simulink model "F550_waypoint"  (R2024a)
settings: Solver=ode4  StartTime=0.0  StopTime=50  FixedStep=Ts  RelTol=1e-3
values from neighbouring files (symbols this model uses):
  armLength = 0.275    [F550_data.m]
  Cd = 0.055    [F550_data.m]
  Cmd = [0.0035 0.0039 0.0034]    [F550_data.m]
  dzcg = 0.12    [F550_data.m]
  g = 9.81    [F550_data.m]
  Inertia = [Jxx, 0, 0;     0, Jyy, 0;     0, 0, Jzz]    [F550_data.m]
  Inertia_inv = inv(Inertia)    [F550_data.m]
  Kd_theta = 1    [sim_F550_waypoint.m]
  Ki_h = 0    [sim_F550_waypoint.m]
  Ki_psi = 0    [sim_F550_waypoint.m]
  Ki_u = 0.02    [sim_F550_waypoint.m]
  Ki_vs = 0.01    [sim_F550_waypoint.m]
  Kp_h = 0.1    [sim_F550_waypoint.m]
  Kp_psi = 1.6    [sim_F550_waypoint.m]
  Kp_r = 0.15    [sim_F550_waypoint.m]
  Kp_theta = 5    [sim_F550_waypoint.m]
  Kp_u = 0.2    [sim_F550_waypoint.m]
  Kp_vs = 0.1    [sim_F550_waypoint.m]
  Mass = 2.06    [F550_data.m]
  motorCr = 1148    [F550_data.m]
  motorJm = 0.0001287    [F550_data.m]
  motorRpm0 = [4000 4000 4000 4000 4000 4000]    [F550_data.m]
  motorTm = 0.02    [F550_data.m]
  motorWb = -141.4    [F550_data.m]
  rotorCm = 1.779e-07    [F550_data.m]
  rotorCt = 1.105e-05    [F550_data.m]
  u0 = opreport.inputs.u    [trim_F550_model.m]
  wp_alt = [100 120 150  80  80]    [sim_F550_waypoint.m]
  wp_east = [0   400 500 500   0]    [sim_F550_waypoint.m]
  wp_north = [100 100 300 500 300]    [sim_F550_waypoint.m]
  wp_u = [  3   5   5   4   3]    [sim_F550_waypoint.m]
  x0 = [0 0 0 0 0 0 0 0 0 0 0 -500]    [F550_data.m]    (also in trim_F550_model.m = opreport.states(7).x)
libraries: matrix_library x2
settings Model: Creator=ADMIN  LastModifiedBy=CNU_UASG
settings DataIOCC: ReturnWorkspaceOutputs=off
settings DebuggingCC: UnconnectedInputMsg=warning  UnconnectedOutputMsg=warning  UnconnectedLineMsg=warning
settings ModelReferenceCC: EnableRefExpFcnMdlSchedulingChecks=on
settings RTWCC: GPUComputeCapability=3.5  DLArmComputeVersion=19.05

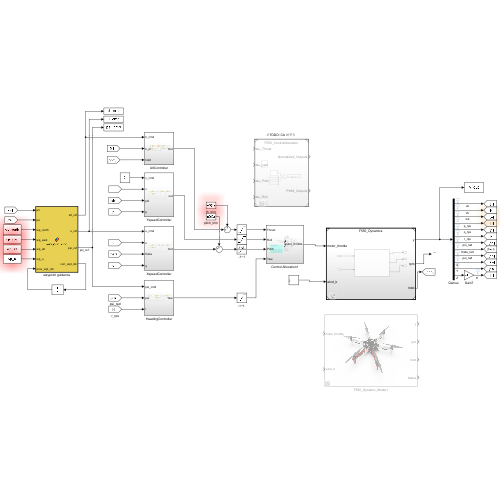
[thumbnail: Simulink's stored preview of the top-level diagram]
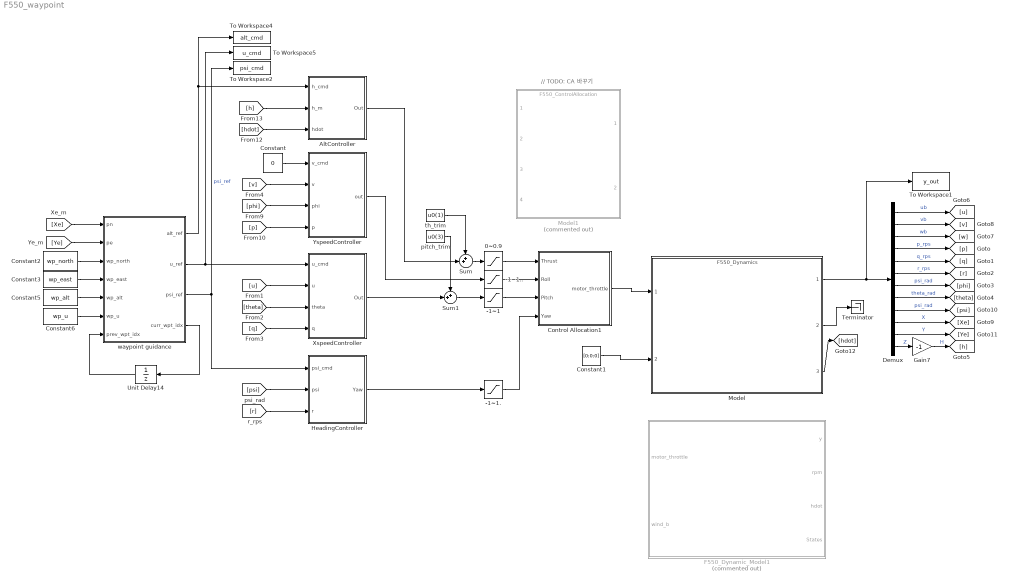
== system F550_waypoint ==
  note: // TODO: CA 바꾸기
  -1~1 : Saturate  UpperLimit=1  LowerLimit=-1
  -1~1. : Saturate  UpperLimit=1  LowerLimit=-1
  -1~1.. : Saturate  UpperLimit=1  LowerLimit=-1
  0~0.9 : Saturate  UpperLimit=0.9  LowerLimit=0
  AltController : Subsystem
  Constant : Constant  Value=0
  Constant1 : Constant  Value=[0;0;0]
  Constant2 : Constant  Value=wp_north  OutDataTypeStr=double
  Constant3 : Constant  Value=wp_east  OutDataTypeStr=double
  Constant5 : Constant  Value=wp_alt  OutDataTypeStr=double
  Constant6 : Constant  Value=wp_u  OutDataTypeStr=double
  Control Allocation1 : Subsystem
  Demux : Demux  Outputs=12
  F550_Dynamic_Model1 : Subsystem  Commented=on
      mask Display: image('F550.jpg');
  Gain7 : Gain  Gain=-1
  HeadingController : Subsystem
  Model : ModelReference  ModelNameDialog=F550_Dynamics.slx  SimulationMode=Normal  ModelReferenceVersion=1.4
  Model1 : ModelReference  Commented=on  ModelNameDialog=F550_ControlAllocation.slx  SimulationMode=Normal  ModelReferenceVersion=1.2
  Sum : Sum  Inputs=++|
  Sum1 : Sum  Inputs=++|
  Terminator : Terminator
  To Workspace1 : ToWorkspace  VariableName=y_out  SampleTime=-1
  To Workspace2 : ToWorkspace  VariableName=psi_cmd  SampleTime=-1
  To Workspace4 : ToWorkspace  VariableName=alt_cmd  SampleTime=-1
  To Workspace5 : ToWorkspace  VariableName=u_cmd  SampleTime=-1
  Unit Delay14 : UnitDelay  InitialCondition=1  SampleTime=-1  HasFrameUpgradeWarning=on
  XspeedController : Subsystem
  YspeedController : Subsystem
  pitch_trim : Constant  Value=u0(3)  OutDataTypeStr=double
  th_trim : Constant  Value=u0(1)  OutDataTypeStr=double
  waypoint guidance : MATLAB Function  TreatAsAtomicUnit=on
  wires:
  th_trim/1 -> Sum/1
  AltController/1(Out) -> Sum/2
  Sum/1 -> 0~0.9/1
  YspeedController/1(out) -> -1~1../1
  Demux/2 -> [v]  "vb"
  Demux/6 -> [r]  "r_rps"
  Demux/8 -> [theta]  "theta_rad"
  Gain7/1 -> [h]  "H"
  Demux/12 -> Gain7/1  "Z"
  Demux/5 -> [q]  "q_rps"
  Demux/3 -> [w]  "wb"
  Demux/4 -> [p]  "p_rps"
  Demux/7 -> [phi]  "psi_rad"
  Demux/1 -> [u]  "ub"
  Model/1 -> To Workspace1/1, Demux/1
  Demux/10 -> [Xe]  "X"
  Demux/11 -> [Ye]  "Y"
  0~0.9/1 -> Control Allocation1/1(Thrust)
  Demux/9 -> [psi]  "psi_rad"
  Constant3/1 -> waypoint guidance/4(wp_east)
  Constant2/1 -> waypoint guidance/3(wp_north)
  waypoint guidance/4(curr_wpt_idx) -> Unit Delay14/1
  Unit Delay14/1 -> waypoint guidance/7(prev_wpt_idx)
  [q] -> XspeedController/4(q)
  [theta] -> XspeedController/3(theta)
  [u] -> XspeedController/2(u)
  waypoint guidance/1(alt_ref) -> AltController/1(h_cmd), To Workspace4/1
  [h] -> AltController/2(h_m)
  [hdot] -> AltController/3(hdot)
  waypoint guidance/3(psi_ref) -> HeadingController/1(psi_cmd), To Workspace2/1  "psi_ref"
  [psi] -> HeadingController/2(psi)
  [r] -> HeadingController/3(r)
  [Ye] -> waypoint guidance/2(pe)
  [Xe] -> waypoint guidance/1(pn)
  Control Allocation1/1(motor_throttle) -> Model/1
  Constant1/1 -> Model/2
  Model/2 -> Terminator/1
  Model/3 -> [hdot]
  Sum1/1 -> -1~1/1
  pitch_trim/1 -> Sum1/1
  XspeedController/1(Out) -> Sum1/2
  -1~1/1 -> Control Allocation1/3(Pitch)
  -1~1./1 -> Control Allocation1/4(Yaw)
  HeadingController/1(Yaw) -> -1~1./1
  Constant/1 -> YspeedController/1(v_cmd)
  [v] -> YspeedController/2(v)
  [phi] -> YspeedController/3(phi)
  [p] -> YspeedController/4(p)
  -1~1../1 -> Control Allocation1/2(Roll)
  Constant5/1 -> waypoint guidance/5(wp_alt)
  Constant6/1 -> waypoint guidance/6(wp_u)
  waypoint guidance/2(u_ref) -> XspeedController/1(u_cmd), To Workspace5/1

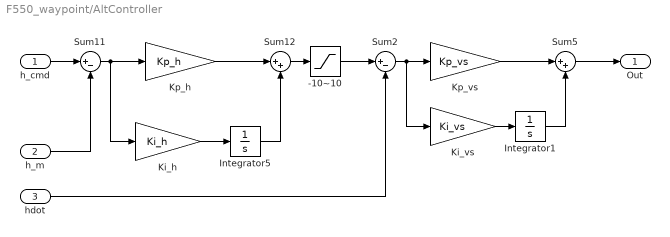
== system F550_waypoint/AltController ==
  h_cmd : Inport
  h_m : Inport  Port=2
  hdot : Inport  Port=3
  -10~10 : Saturate  UpperLimit=10  LowerLimit=-10
  Integrator1 : Integrator
  Integrator5 : Integrator
  Ki_h : Gain  Gain=Ki_h  SaturateOnIntegerOverflow=on  OutDataTypeStr=Inherit: Same as input  ParamDataTypeStr=Inherit: Same as input
  Ki_vs : Gain  Gain=Ki_vs  SaturateOnIntegerOverflow=on  OutDataTypeStr=Inherit: Same as input  ParamDataTypeStr=Inherit: Same as input
  Kp_h : Gain  Gain=Kp_h  SaturateOnIntegerOverflow=on  OutDataTypeStr=Inherit: Same as input  ParamDataTypeStr=Inherit: Same as input
  Kp_vs : Gain  Gain=Kp_vs  SaturateOnIntegerOverflow=on  OutDataTypeStr=Inherit: Same as input  ParamDataTypeStr=Inherit: Same as input
  Sum11 : Sum  Inputs=|+-  InputSameDT=on  SaturateOnIntegerOverflow=on  OutDataTypeStr=Inherit: Same as first input
  Sum12 : Sum  Inputs=|++  InputSameDT=on  SaturateOnIntegerOverflow=on  OutDataTypeStr=Inherit: Same as first input
  Sum2 : Sum  Inputs=|+-  InputSameDT=on  SaturateOnIntegerOverflow=on  OutDataTypeStr=Inherit: Same as first input
  Sum5 : Sum  Inputs=|++  InputSameDT=on  SaturateOnIntegerOverflow=on  OutDataTypeStr=Inherit: Same as first input
  Out : Outport
  wires:
  -10~10/1 -> Sum2/1
  Sum11/1 -> Kp_h/1, Ki_h/1
  Kp_vs/1 -> Sum5/1
  Sum12/1 -> -10~10/1
  Integrator1/1 -> Sum5/2
  Sum2/1 -> Kp_vs/1, Ki_vs/1
  Integrator5/1 -> Sum12/2
  Ki_h/1 -> Integrator5/1
  Kp_h/1 -> Sum12/1
  Ki_vs/1 -> Integrator1/1
  Sum5/1 -> Out/1
  h_m/1 -> Sum11/2
  h_cmd/1 -> Sum11/1
  hdot/1 -> Sum2/2

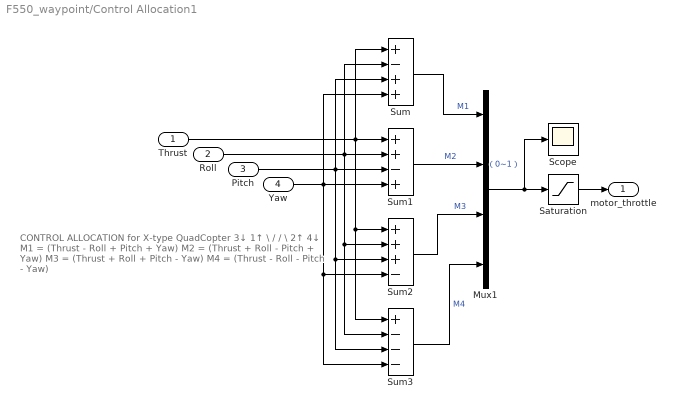
== system F550_waypoint/Control Allocation1 ==
  note: CONTROL ALLOCATION
      | for X-type QuadCopter
      | 3↓ 1↑
      | \ /
      | / \
      | 2↑ 4↓
      | M1 = (Thrust - Roll + Pitch + Yaw)
      | M2 = (Thrust + Roll - Pitch + Yaw)
      | M3 = (Thrust + Roll + Pitch - Yaw)
      | M4 = (Thrust - Roll - Pitch - Yaw)
  Thrust : Inport
  Roll : Inport  Port=2
  Pitch : Inport  Port=3
  Yaw : Inport  Port=4
  Mux1 : Mux
  Saturation : Saturate  UpperLimit=1  LowerLimit=0
  Scope : Scope
  Sum : Sum  Inputs=+-++
  Sum1 : Sum  Inputs=++-+
  Sum2 : Sum  Inputs=+++-
  Sum3 : Sum  Inputs=+---
  motor_throttle : Outport
  wires:
  Thrust/1 -> Sum3/1, Sum2/1, Sum/1, Sum1/1
  Sum3/1 -> Mux1/4  "M4"
  Sum1/1 -> Mux1/2  "M2"
  Yaw/1 -> Sum3/4, Sum2/4, Sum/4, Sum1/4
  Sum/1 -> Mux1/1  "M1"
  Roll/1 -> Sum3/2, Sum2/2, Sum/2, Sum1/2
  Sum2/1 -> Mux1/3  "M3"
  Mux1/1 -> Scope/1, Saturation/1  "（0~1）"
  Pitch/1 -> Sum3/3, Sum2/3, Sum/3, Sum1/3
  Saturation/1 -> motor_throttle/1

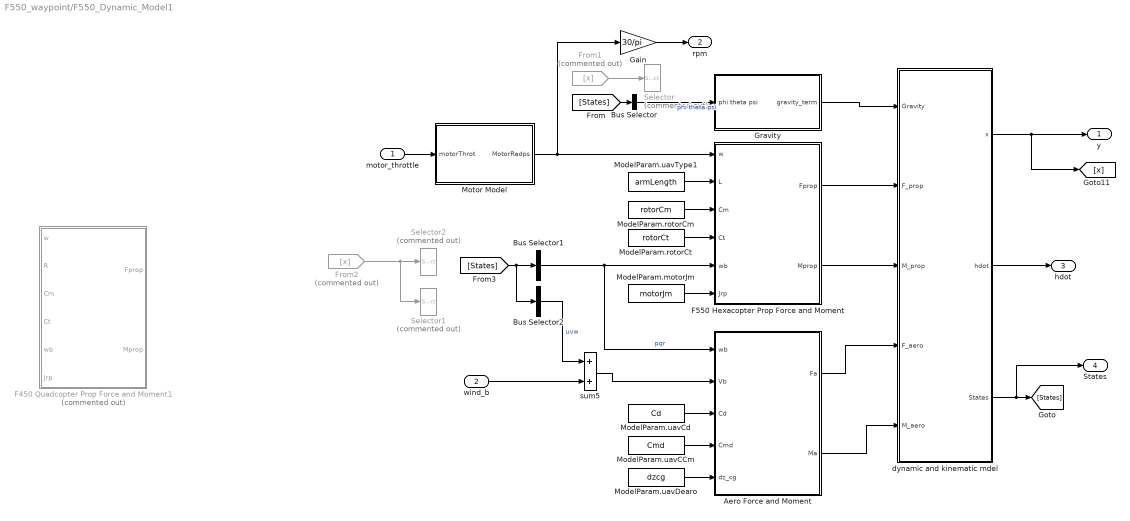
== system F550_waypoint/F550_Dynamic_Model1 ==
  motor_throttle : Inport
  wind_b : Inport  Port=2
  Aero Force and Moment : MATLAB Function  TreatAsAtomicUnit=on
  Bus Selector : BusSelector  OutputSignals=Phi,Theta,Psi  OutputAsBus=on
  Bus Selector1 : BusSelector  OutputSignals=P,Q,R  OutputAsBus=on
  Bus Selector2 : BusSelector  OutputSignals=U,V,W  OutputAsBus=on
  F450 Quadcopter Prop Force and Moment1 : MATLAB Function  Commented=on  TreatAsAtomicUnit=on
  F550 Hexacopter Prop Force and Moment : MATLAB Function  TreatAsAtomicUnit=on
  From1 : From  Commented=on  GotoTag=x
  From2 : From  Commented=on  GotoTag=x
  Gain : Gain  Gain=30/pi
  Gravity : Subsystem
  ModelParam.motorJm : Constant  Value=motorJm
  ModelParam.rotorCm : Constant  Value=rotorCm
  ModelParam.rotorCt : Constant  Value=rotorCt
  ModelParam.uavCCm : Constant  Value=Cmd
  ModelParam.uavCd : Constant  Value=Cd
  ModelParam.uavDearo : Constant  Value=dzcg
  ModelParam.uavType1 : Constant  Value=armLength
  Motor Model : Subsystem
  Selector : Selector  Commented=on  InputPortWidth=12  IndexOptions=Index vector (dialog)  Indices=[7 8 9]  OutputSizes=1
  Selector1 : Selector  Commented=on  InputPortWidth=12  IndexOptions=Index vector (dialog)  Indices=[1 2 3]  OutputSizes=1
  Selector2 : Selector  Commented=on  InputPortWidth=12  IndexOptions=Index vector (dialog)  Indices=[4 5 6]  OutputSizes=1
  dynamic and kinematic mdel : Subsystem
  sum5 : Sum  InputSameDT=on  SaturateOnIntegerOverflow=on  OutDataTypeStr=Inherit: Same as first input
  y : Outport
  rpm : Outport  Port=2
  hdot : Outport  Port=3
  States : Outport  Port=4
  wires:
  ModelParam.uavDearo/1 -> Aero Force and Moment/5(dz_cg)
  ModelParam.uavCCm/1 -> Aero Force and Moment/4(Cmd)
  ModelParam.uavCd/1 -> Aero Force and Moment/3(Cd)
  Aero Force and Moment/2(Ma) -> dynamic and kinematic mdel/5(M_aero)
  Aero Force and Moment/1(Fa) -> dynamic and kinematic mdel/4(F_aero)
  F550 Hexacopter Prop Force and Moment/2(Mprop) -> dynamic and kinematic mdel/3(M_prop)
  F550 Hexacopter Prop Force and Moment/1(Fprop) -> dynamic and kinematic mdel/2(F_prop)
  ModelParam.motorJm/1 -> F550 Hexacopter Prop Force and Moment/6(Jrp)
  ModelParam.uavType1/1 -> F550 Hexacopter Prop Force and Moment/2(L)
  ModelParam.rotorCt/1 -> F550 Hexacopter Prop Force and Moment/4(Ct)
  ModelParam.rotorCm/1 -> F550 Hexacopter Prop Force and Moment/3(Cm)
  Gravity/1(gravity_term) -> dynamic and kinematic mdel/1(Gravity)
  motor_throttle/1 -> Motor Model/1(motorThrot)
  Gain/1 -> rpm/1
  From1/1 -> Selector/1
  From2/1 -> Selector2/1, Selector1/1
  Motor Model/1(MotorRadps) -> F550 Hexacopter Prop Force and Moment/1(w), Gain/1
  wind_b/1 -> sum5/2
  sum5/1 -> Aero Force and Moment/2(Vb)
  dynamic and kinematic mdel/1(x) -> y/1, [x]
  dynamic and kinematic mdel/2(hdot) -> hdot/1
  dynamic and kinematic mdel/3(States) -> States/1, [States]
  [States] -> Bus Selector/1
  Bus Selector/1 -> Gravity/1(phi theta psi)  "phi theta psi"
  [States] -> Bus Selector2/1, Bus Selector1/1
  Bus Selector1/1 -> Aero Force and Moment/1(wb), F550 Hexacopter Prop Force and Moment/5(wb)  "pqr"
  Bus Selector2/1 -> sum5/1  "uvw"

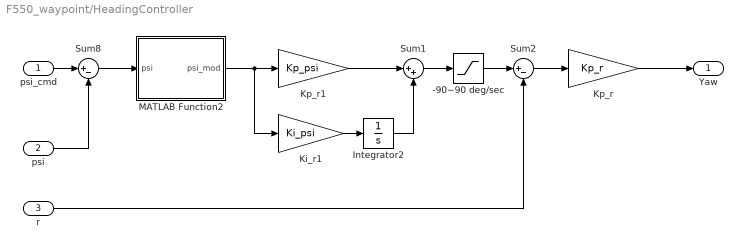
== system F550_waypoint/HeadingController ==
  psi_cmd : Inport
  psi : Inport  Port=2
  r : Inport  Port=3
  -90~90 deg/sec : Saturate  UpperLimit=90/57.3  LowerLimit=-90/57.3
  Integrator2 : Integrator
  Ki_r1 : Gain  Gain=Ki_psi  SaturateOnIntegerOverflow=on  OutDataTypeStr=Inherit: Same as input  ParamDataTypeStr=Inherit: Same as input
  Kp_r : Gain  Gain=Kp_r  SaturateOnIntegerOverflow=on  OutDataTypeStr=Inherit: Same as input  ParamDataTypeStr=Inherit: Same as input
  Kp_r1 : Gain  Gain=Kp_psi  SaturateOnIntegerOverflow=on  OutDataTypeStr=Inherit: Same as input  ParamDataTypeStr=Inherit: Same as input
  MATLAB Function2 : MATLAB Function  TreatAsAtomicUnit=on
  Sum1 : Sum  Inputs=|++  InputSameDT=on  SaturateOnIntegerOverflow=on  OutDataTypeStr=Inherit: Same as first input
  Sum2 : Sum  Inputs=|+-  InputSameDT=on  SaturateOnIntegerOverflow=on  OutDataTypeStr=Inherit: Same as first input
  Sum8 : Sum  Inputs=|+-  InputSameDT=on  SaturateOnIntegerOverflow=on  OutDataTypeStr=Inherit: Same as first input
  Yaw : Outport
  wires:
  Sum2/1 -> Kp_r/1
  Sum1/1 -> -90~90 deg/sec/1
  Kp_r1/1 -> Sum1/1
  Kp_r/1 -> Yaw/1
  Ki_r1/1 -> Integrator2/1
  Integrator2/1 -> Sum1/2
  -90~90 deg/sec/1 -> Sum2/1
  r/1 -> Sum2/2
  psi/1 -> Sum8/2
  psi_cmd/1 -> Sum8/1
  Sum8/1 -> MATLAB Function2/1(psi)
  MATLAB Function2/1(psi_mod) -> Kp_r1/1, Ki_r1/1

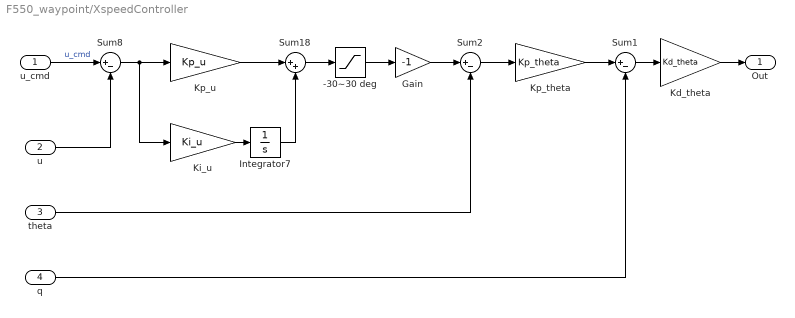
== system F550_waypoint/XspeedController ==
  u_cmd : Inport
  u : Inport  Port=2
  theta : Inport  Port=3
  q : Inport  Port=4
  -30~30 deg : Saturate  UpperLimit=30/57.3  LowerLimit=-30/57.3
  Gain : Gain  Gain=-1
  Integrator7 : Integrator
  Kd_theta : Gain  Gain=Kd_theta  SaturateOnIntegerOverflow=on  OutDataTypeStr=Inherit: Same as input  ParamDataTypeStr=Inherit: Same as input
  Ki_u : Gain  Gain=Ki_u  SaturateOnIntegerOverflow=on  OutDataTypeStr=Inherit: Same as input  ParamDataTypeStr=Inherit: Same as input
  Kp_theta : Gain  Gain=Kp_theta  SaturateOnIntegerOverflow=on  OutDataTypeStr=Inherit: Same as input  ParamDataTypeStr=Inherit: Same as input
  Kp_u : Gain  Gain=Kp_u  SaturateOnIntegerOverflow=on  OutDataTypeStr=Inherit: Same as input  ParamDataTypeStr=Inherit: Same as input
  Sum1 : Sum  Inputs=|+-  InputSameDT=on  SaturateOnIntegerOverflow=on  OutDataTypeStr=Inherit: Same as first input
  Sum18 : Sum  Inputs=|++  InputSameDT=on  SaturateOnIntegerOverflow=on  OutDataTypeStr=Inherit: Same as first input
  Sum2 : Sum  Inputs=|+-  InputSameDT=on  SaturateOnIntegerOverflow=on  OutDataTypeStr=Inherit: Same as first input
  Sum8 : Sum  Inputs=|+-  InputSameDT=on  SaturateOnIntegerOverflow=on  OutDataTypeStr=Inherit: Same as first input
  Out : Outport
  wires:
  -30~30 deg/1 -> Gain/1
  Kp_u/1 -> Sum18/1
  Sum2/1 -> Kp_theta/1
  Ki_u/1 -> Integrator7/1
  Sum18/1 -> -30~30 deg/1
  theta/1 -> Sum2/2
  Sum8/1 -> Ki_u/1, Kp_u/1
  Gain/1 -> Sum2/1
  q/1 -> Sum1/2
  Integrator7/1 -> Sum18/2
  Kp_theta/1 -> Sum1/1
  u_cmd/1 -> Sum8/1  "u_cmd"
  Sum1/1 -> Kd_theta/1
  u/1 -> Sum8/2
  Kd_theta/1 -> Out/1

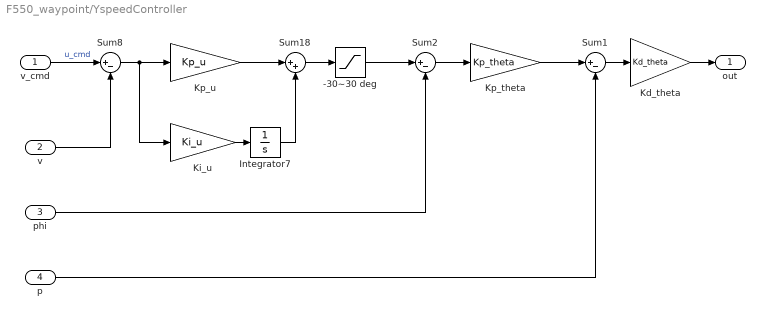
== system F550_waypoint/YspeedController ==
  v_cmd : Inport
  v : Inport  Port=2
  phi : Inport  Port=3
  p : Inport  Port=4
  -30~30 deg : Saturate  UpperLimit=30/57.3  LowerLimit=-30/57.3
  Integrator7 : Integrator
  Kd_theta : Gain  Gain=Kd_theta  SaturateOnIntegerOverflow=on  OutDataTypeStr=Inherit: Same as input  ParamDataTypeStr=Inherit: Same as input
  Ki_u : Gain  Gain=Ki_u  SaturateOnIntegerOverflow=on  OutDataTypeStr=Inherit: Same as input  ParamDataTypeStr=Inherit: Same as input
  Kp_theta : Gain  Gain=Kp_theta  SaturateOnIntegerOverflow=on  OutDataTypeStr=Inherit: Same as input  ParamDataTypeStr=Inherit: Same as input
  Kp_u : Gain  Gain=Kp_u  SaturateOnIntegerOverflow=on  OutDataTypeStr=Inherit: Same as input  ParamDataTypeStr=Inherit: Same as input
  Sum1 : Sum  Inputs=|+-  InputSameDT=on  SaturateOnIntegerOverflow=on  OutDataTypeStr=Inherit: Same as first input
  Sum18 : Sum  Inputs=|++  InputSameDT=on  SaturateOnIntegerOverflow=on  OutDataTypeStr=Inherit: Same as first input
  Sum2 : Sum  Inputs=|+-  InputSameDT=on  SaturateOnIntegerOverflow=on  OutDataTypeStr=Inherit: Same as first input
  Sum8 : Sum  Inputs=|+-  InputSameDT=on  SaturateOnIntegerOverflow=on  OutDataTypeStr=Inherit: Same as first input
  out : Outport
  wires:
  Kd_theta/1 -> out/1
  v/1 -> Sum8/2
  Sum1/1 -> Kd_theta/1
  v_cmd/1 -> Sum8/1  "u_cmd"
  Kp_theta/1 -> Sum1/1
  Integrator7/1 -> Sum18/2
  p/1 -> Sum1/2
  Sum8/1 -> Kp_u/1, Ki_u/1
  phi/1 -> Sum2/2
  Sum18/1 -> -30~30 deg/1
  Ki_u/1 -> Integrator7/1
  Sum2/1 -> Kp_theta/1
  Kp_u/1 -> Sum18/1
  -30~30 deg/1 -> Sum2/1

== system F550_waypoint/F550_Dynamic_Model1/Gravity ==
  note: Gravaity
  phi theta psi : Inport
  . : Gain  Gain=g*Mass  SaturateOnIntegerOverflow=on  OutDataTypeStr=Inherit: Same as input  ParamDataTypeStr=Inherit: Same as input
  Mux : Mux  Inputs=3
  psidot2 : Fcn  Expr=cos(u[2])*cos(u[1])
  t : Fcn  Expr=-sin(u[2])
  tetadot : Fcn  Expr=cos(u[2])*sin(u[1])
  gravity_term : Outport  InitialOutput=0  VectorParamsAs1DForOutWhenUnconnected=off
  wires:
  t/1 -> Mux/1
  psidot2/1 -> Mux/3
  tetadot/1 -> Mux/2
  Mux/1 -> ./1
  phi theta psi/1 -> tetadot/1, t/1, psidot2/1
  ./1 -> gravity_term/1

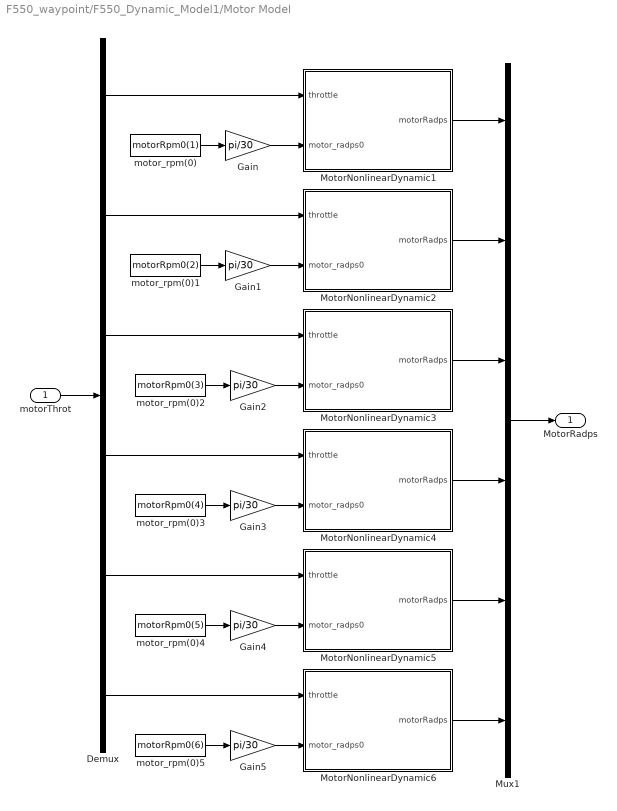
== system F550_waypoint/F550_Dynamic_Model1/Motor Model ==
  motorThrot : Inport
  Demux : Demux  Outputs=6
  Gain{,1..5} (6 alike) : Gain  Gain=pi/30
  MotorNonlinearDynamic1 : Subsystem  TreatAsAtomicUnit=on
  MotorNonlinearDynamic2 : Subsystem  TreatAsAtomicUnit=on
  MotorNonlinearDynamic3 : Subsystem  TreatAsAtomicUnit=on
  MotorNonlinearDynamic4 : Subsystem  TreatAsAtomicUnit=on
  MotorNonlinearDynamic5 : Subsystem  TreatAsAtomicUnit=on
  MotorNonlinearDynamic6 : Subsystem  TreatAsAtomicUnit=on
  Mux1 : Mux  Inputs=6
  motor_rpm(0) : Constant  Value=motorRpm0(1)
  motor_rpm(0)1 : Constant  Value=motorRpm0(2)
  motor_rpm(0)2 : Constant  Value=motorRpm0(3)
  motor_rpm(0)3 : Constant  Value=motorRpm0(4)
  motor_rpm(0)4 : Constant  Value=motorRpm0(5)
  motor_rpm(0)5 : Constant  Value=motorRpm0(6)
  MotorRadps : Outport  VectorParamsAs1DForOutWhenUnconnected=off
  wires:
  motorThrot/1 -> Demux/1
  Demux/4 -> MotorNonlinearDynamic4/1(throttle)
  motor_rpm(0)/1 -> Gain/1
  MotorNonlinearDynamic3/1(motorRadps) -> Mux1/3
  MotorNonlinearDynamic2/1(motorRadps) -> Mux1/2
  Mux1/1 -> MotorRadps/1
  Demux/2 -> MotorNonlinearDynamic2/1(throttle)
  Demux/3 -> MotorNonlinearDynamic3/1(throttle)
  Demux/1 -> MotorNonlinearDynamic1/1(throttle)
  MotorNonlinearDynamic4/1(motorRadps) -> Mux1/4
  MotorNonlinearDynamic1/1(motorRadps) -> Mux1/1
  Gain/1 -> MotorNonlinearDynamic1/2(motor_radps0)
  motor_rpm(0)1/1 -> Gain1/1
  Gain1/1 -> MotorNonlinearDynamic2/2(motor_radps0)
  motor_rpm(0)2/1 -> Gain2/1
  Gain2/1 -> MotorNonlinearDynamic3/2(motor_radps0)
  motor_rpm(0)3/1 -> Gain3/1
  Gain3/1 -> MotorNonlinearDynamic4/2(motor_radps0)
  Gain4/1 -> MotorNonlinearDynamic5/2(motor_radps0)
  motor_rpm(0)4/1 -> Gain4/1
  Demux/5 -> MotorNonlinearDynamic5/1(throttle)
  Gain5/1 -> MotorNonlinearDynamic6/2(motor_radps0)
  motor_rpm(0)5/1 -> Gain5/1
  Demux/6 -> MotorNonlinearDynamic6/1(throttle)
  MotorNonlinearDynamic5/1(motorRadps) -> Mux1/5
  MotorNonlinearDynamic6/1(motorRadps) -> Mux1/6

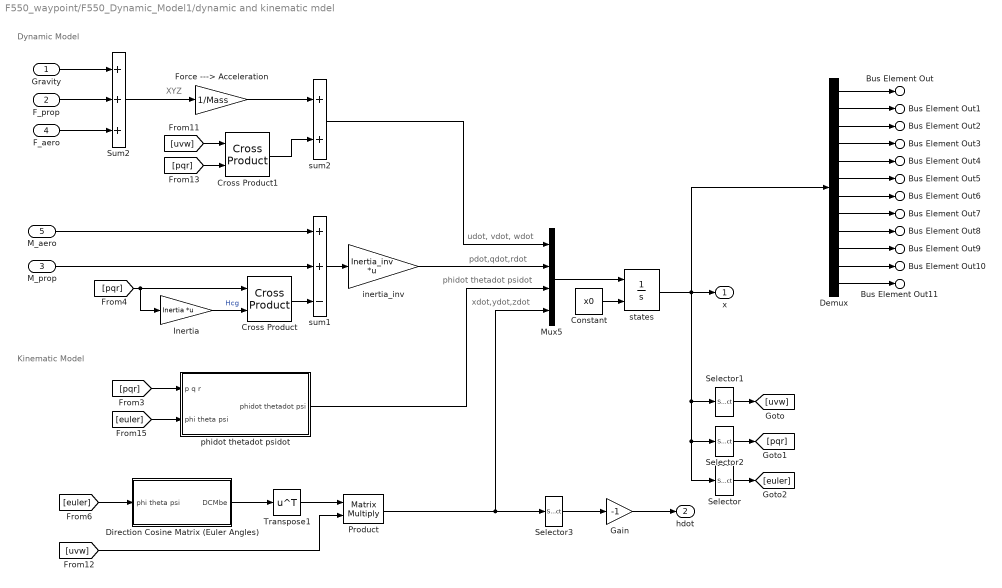
== system F550_waypoint/F550_Dynamic_Model1/dynamic and kinematic mdel ==
  note: Kinematic Model
  note: udot, vdot, wdot
  note: pdot,qdot,rdot
  note: phidot thetadot psidot
  note: xdot,ydot,zdot
  note: XYZ
  note: Dynamic Model
  Gravity : Inport
  F_prop : Inport  Port=2
  M_prop : Inport  Port=3
  F_aero : Inport  Port=4
  M_aero : Inport  Port=5
  Constant : Constant  Value=x0
  Cross Product : matrix_library/Cross Product
  Cross Product1 : matrix_library/Cross Product
  Demux : Demux  Outputs=12
  Direction Cosine Matrix (Euler Angles) : Subsystem
  Force ---> Acceleration : Gain  Gain=1/Mass  SaturateOnIntegerOverflow=on  OutDataTypeStr=Inherit: Same as input  ParamDataTypeStr=Inherit: Same as input
  Gain : Gain  Gain=-1
  Inertia : Gain  Gain=Inertia  Multiplication=Matrix(K*u)
  Mux5 : Mux
  Product : Product  Multiplication=Matrix(*)  InputSameDT=on  RndMeth=Zero  SaturateOnIntegerOverflow=on  OutDataTypeStr=Inherit: Same as first input
  Selector : Selector  InputPortWidth=12  IndexOptions=Index vector (dialog)  Indices=[7 8 9]  OutputSizes=1
  Selector1 : Selector  InputPortWidth=12  IndexOptions=Index vector (dialog)  Indices=[1 2 3]  OutputSizes=1
  Selector2 : Selector  InputPortWidth=12  IndexOptions=Index vector (dialog)  Indices=[4 5 6]  OutputSizes=1
  Selector3 : Selector  InputPortWidth=3  IndexOptions=Index vector (dialog)  Indices=3  OutputSizes=1
  Sum2 : Sum  Inputs=+++  InputSameDT=on  SaturateOnIntegerOverflow=on  OutDataTypeStr=Inherit: Same as first input
  Transpose1 : Math  Operator=transpose  SignedPower=on
  inertia_inv : Gain  Gain=Inertia_inv  Multiplication=Matrix(K*u)
  phidot thetadot psidot : Subsystem
  states : Integrator  InitialConditionSource=external  InitialCondition=x0
  sum1 : Sum  Inputs=++-  InputSameDT=on  SaturateOnIntegerOverflow=on  OutDataTypeStr=Inherit: Same as first input
  sum2 : Sum  InputSameDT=on  SaturateOnIntegerOverflow=on  OutDataTypeStr=Inherit: Same as first input
  x : Outport  VectorParamsAs1DForOutWhenUnconnected=off
  hdot : Outport  Port=2  VectorParamsAs1DForOutWhenUnconnected=off
  Bus Element Out : Outport  Port=3  PortName=States  Element=U
  Bus Element Out1 : Outport  Port=3  PortName=States  Element=V
  Bus Element Out2 : Outport  Port=3  PortName=States  Element=W
  Bus Element Out3 : Outport  Port=3  PortName=States  Element=P
  Bus Element Out4 : Outport  Port=3  PortName=States  Element=Q
  Bus Element Out5 : Outport  Port=3  PortName=States  Element=R
  Bus Element Out6 : Outport  Port=3  PortName=States  Element=Phi
  Bus Element Out7 : Outport  Port=3  PortName=States  Element=Theta
  Bus Element Out8 : Outport  Port=3  PortName=States  Element=Psi
  Bus Element Out9 : Outport  Port=3  PortName=States  Element=X
  Bus Element Out10 : Outport  Port=3  PortName=States  Element=Y
  Bus Element Out11 : Outport  Port=3  PortName=States  Element=Z
  wires:
  [euler] -> Direction Cosine Matrix (Euler Angles)/1(phi theta psi)
  [uvw] -> Product/2
  Direction Cosine Matrix (Euler Angles)/1(DCMbe) -> Transpose1/1
  Transpose1/1 -> Product/1
  Gravity/1 -> Sum2/1
  M_prop/1 -> sum1/2
  Cross Product/1 -> sum1/3
  M_aero/1 -> sum1/1
  F_aero/1 -> Sum2/3
  F_prop/1 -> Sum2/2
  Sum2/1 -> Force ---> Acceleration/1
  Force ---> Acceleration/1 -> sum2/1
  Cross Product1/1 -> sum2/2
  sum1/1 -> inertia_inv/1
  Inertia/1 -> Cross Product/2  "Hcg"
  phidot thetadot psidot/1(phidot thetadot psi) -> Mux5/3
  sum2/1 -> Mux5/1
  inertia_inv/1 -> Mux5/2
  Mux5/1 -> states/1
  [pqr] -> Inertia/1, Cross Product/1
  [uvw] -> Cross Product1/1
  [pqr] -> Cross Product1/2
  [euler] -> phidot thetadot psidot/2(phi theta psi)
  Product/1 -> Selector3/1, Mux5/4
  [pqr] -> phidot thetadot psidot/1(p q r)
  Selector2/1 -> [pqr]
  states/1 -> Demux/1, Selector1/1, Selector/1, Selector2/1, x/1
  Selector1/1 -> [uvw]
  Constant/1 -> states/2
  Selector/1 -> [euler]
  Selector3/1 -> Gain/1
  Gain/1 -> hdot/1
  Demux/1 -> Bus Element Out/1
  Demux/2 -> Bus Element Out1/1
  Demux/3 -> Bus Element Out2/1
  Demux/5 -> Bus Element Out4/1
  Demux/4 -> Bus Element Out3/1
  Demux/6 -> Bus Element Out5/1
  Demux/7 -> Bus Element Out6/1
  Demux/8 -> Bus Element Out7/1
  Demux/9 -> Bus Element Out8/1
  Demux/10 -> Bus Element Out9/1
  Demux/11 -> Bus Element Out10/1
  Demux/12 -> Bus Element Out11/1

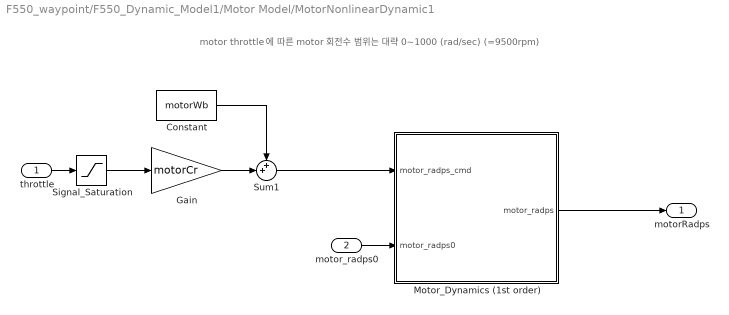
== system F550_waypoint/F550_Dynamic_Model1/Motor Model/MotorNonlinearDynamic1 ==
  note: motor throttle 에 따른 motor 회전수 범위는 대략 0~1000 (rad/sec) (=9500rpm)
  throttle : Inport
  motor_radps0 : Inport  Port=2
  Constant : Constant  Value=motorWb
  Gain : Gain  Gain=motorCr
  Motor_Dynamics (1st order) : Subsystem  TreatAsAtomicUnit=on
  Signal_Saturation : Saturate  UpperLimit=0.95  LowerLimit=0
      settings: AttributesFormatString=%<LowerLimit>~%<UpperLimit>
  Sum1 : Sum  Inputs=++|
  motorRadps : Outport  VectorParamsAs1DForOutWhenUnconnected=off
  wires:
  Motor_Dynamics (1st order)/1(motor_radps) -> motorRadps/1
  motor_radps0/1 -> Motor_Dynamics (1st order)/2(motor_radps0)
  Constant/1 -> Sum1/1
  Gain/1 -> Sum1/2
  Signal_Saturation/1 -> Gain/1
  Sum1/1 -> Motor_Dynamics (1st order)/1(motor_radps_cmd)
  throttle/1 -> Signal_Saturation/1

== system F550_waypoint/F550_Dynamic_Model1/Motor Model/MotorNonlinearDynamic2 ==
  note: motor throttle 에 따른 motor 회전수 범위는 대략 0~1000 (rad/sec) (=9500rpm)
  throttle : Inport
  motor_radps0 : Inport  Port=2
  Constant : Constant  Value=motorWb
  Gain : Gain  Gain=motorCr
  Motor_Dynamics (1st order) : Subsystem  TreatAsAtomicUnit=on
  Signal_Saturation : Saturate  UpperLimit=0.95  LowerLimit=0
      settings: AttributesFormatString=%<LowerLimit>~%<UpperLimit>
  Sum1 : Sum  Inputs=++|
  motorRadps : Outport  VectorParamsAs1DForOutWhenUnconnected=off
  wires:
  throttle/1 -> Signal_Saturation/1
  Sum1/1 -> Motor_Dynamics (1st order)/1(motor_radps_cmd)
  Signal_Saturation/1 -> Gain/1
  Gain/1 -> Sum1/2
  Constant/1 -> Sum1/1
  motor_radps0/1 -> Motor_Dynamics (1st order)/2(motor_radps0)
  Motor_Dynamics (1st order)/1(motor_radps) -> motorRadps/1

== system F550_waypoint/F550_Dynamic_Model1/Motor Model/MotorNonlinearDynamic3 ==
  note: motor throttle 에 따른 motor 회전수 범위는 대략 0~1000 (rad/sec) (=9500rpm)
  throttle : Inport
  motor_radps0 : Inport  Port=2
  Constant : Constant  Value=motorWb
  Gain : Gain  Gain=motorCr
  Motor_Dynamics (1st order) : Subsystem  TreatAsAtomicUnit=on
  Signal_Saturation : Saturate  UpperLimit=0.95  LowerLimit=0
      settings: AttributesFormatString=%<LowerLimit>~%<UpperLimit>
  Sum1 : Sum  Inputs=++|
  motorRadps : Outport  VectorParamsAs1DForOutWhenUnconnected=off
  wires:
  Motor_Dynamics (1st order)/1(motor_radps) -> motorRadps/1
  motor_radps0/1 -> Motor_Dynamics (1st order)/2(motor_radps0)
  Constant/1 -> Sum1/1
  Gain/1 -> Sum1/2
  Signal_Saturation/1 -> Gain/1
  Sum1/1 -> Motor_Dynamics (1st order)/1(motor_radps_cmd)
  throttle/1 -> Signal_Saturation/1

== system F550_waypoint/F550_Dynamic_Model1/Motor Model/MotorNonlinearDynamic4 ==
  note: motor throttle 에 따른 motor 회전수 범위는 대략 0~1000 (rad/sec) (=9500rpm)
  throttle : Inport
  motor_radps0 : Inport  Port=2
  Constant : Constant  Value=motorWb
  Gain : Gain  Gain=motorCr
  Motor_Dynamics (1st order) : Subsystem  TreatAsAtomicUnit=on
  Signal_Saturation : Saturate  UpperLimit=0.95  LowerLimit=0
      settings: AttributesFormatString=%<LowerLimit>~%<UpperLimit>
  Sum1 : Sum  Inputs=++|
  motorRadps : Outport  VectorParamsAs1DForOutWhenUnconnected=off
  wires:
  throttle/1 -> Signal_Saturation/1
  Sum1/1 -> Motor_Dynamics (1st order)/1(motor_radps_cmd)
  Signal_Saturation/1 -> Gain/1
  Gain/1 -> Sum1/2
  Constant/1 -> Sum1/1
  motor_radps0/1 -> Motor_Dynamics (1st order)/2(motor_radps0)
  Motor_Dynamics (1st order)/1(motor_radps) -> motorRadps/1

== system F550_waypoint/F550_Dynamic_Model1/Motor Model/MotorNonlinearDynamic5 ==
  note: motor throttle 에 따른 motor 회전수 범위는 대략 0~1000 (rad/sec) (=9500rpm)
  throttle : Inport
  motor_radps0 : Inport  Port=2
  Constant : Constant  Value=motorWb
  Gain : Gain  Gain=motorCr
  Motor_Dynamics (1st order) : Subsystem  TreatAsAtomicUnit=on
  Signal_Saturation : Saturate  UpperLimit=0.95  LowerLimit=0
      settings: AttributesFormatString=%<LowerLimit>~%<UpperLimit>
  Sum1 : Sum  Inputs=++|
  motorRadps : Outport  VectorParamsAs1DForOutWhenUnconnected=off
  wires:
  throttle/1 -> Signal_Saturation/1
  Sum1/1 -> Motor_Dynamics (1st order)/1(motor_radps_cmd)
  Signal_Saturation/1 -> Gain/1
  Gain/1 -> Sum1/2
  Constant/1 -> Sum1/1
  motor_radps0/1 -> Motor_Dynamics (1st order)/2(motor_radps0)
  Motor_Dynamics (1st order)/1(motor_radps) -> motorRadps/1

== system F550_waypoint/F550_Dynamic_Model1/Motor Model/MotorNonlinearDynamic6 ==
  note: motor throttle 에 따른 motor 회전수 범위는 대략 0~1000 (rad/sec) (=9500rpm)
  throttle : Inport
  motor_radps0 : Inport  Port=2
  Constant : Constant  Value=motorWb
  Gain : Gain  Gain=motorCr
  Motor_Dynamics (1st order) : Subsystem  TreatAsAtomicUnit=on
  Signal_Saturation : Saturate  UpperLimit=0.95  LowerLimit=0
      settings: AttributesFormatString=%<LowerLimit>~%<UpperLimit>
  Sum1 : Sum  Inputs=++|
  motorRadps : Outport  VectorParamsAs1DForOutWhenUnconnected=off
  wires:
  throttle/1 -> Signal_Saturation/1
  Sum1/1 -> Motor_Dynamics (1st order)/1(motor_radps_cmd)
  Signal_Saturation/1 -> Gain/1
  Gain/1 -> Sum1/2
  Constant/1 -> Sum1/1
  motor_radps0/1 -> Motor_Dynamics (1st order)/2(motor_radps0)
  Motor_Dynamics (1st order)/1(motor_radps) -> motorRadps/1

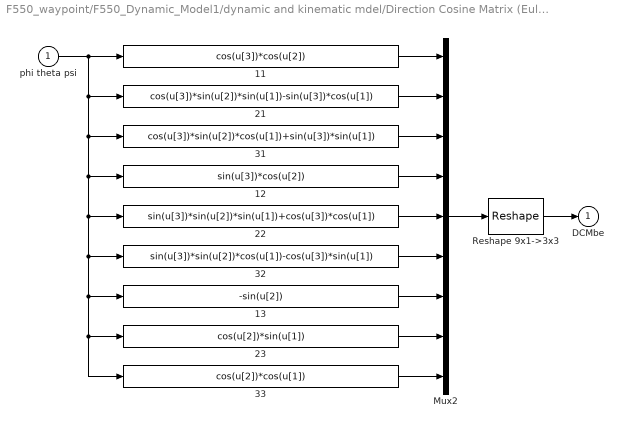
== system F550_waypoint/F550_Dynamic_Model1/dynamic and kinematic mdel/Direction Cosine Matrix (Euler Angles) ==
  phi theta psi : Inport
  11 : Fcn  Expr=cos(u[3])*cos(u[2])
  12 : Fcn  Expr=sin(u[3])*cos(u[2])
  13 : Fcn  Expr=-sin(u[2])
  21 : Fcn  Expr=cos(u[3])*sin(u[2])*sin(u[1])-sin(u[3])*cos(u[1])
  22 : Fcn  Expr=sin(u[3])*sin(u[2])*sin(u[1])+cos(u[3])*cos(u[1])
  23 : Fcn  Expr=cos(u[2])*sin(u[1])
  31 : Fcn  Expr=cos(u[3])*sin(u[2])*cos(u[1])+sin(u[3])*sin(u[1])
  32 : Fcn  Expr=sin(u[3])*sin(u[2])*cos(u[1])-cos(u[3])*sin(u[1])
  33 : Fcn  Expr=cos(u[2])*cos(u[1])
  Mux2 : Mux  Inputs=9
  Reshape 9x1->3x3 : Reshape  OutputDimensionality=Customize  OutputDimensions=[3,3]
  DCMbe : Outport  InitialOutput=0  VectorParamsAs1DForOutWhenUnconnected=off
  wires:
  31/1 -> Mux2/3
  Mux2/1 -> Reshape 9x1->3x3/1
  11/1 -> Mux2/1
  12/1 -> Mux2/4
  13/1 -> Mux2/7
  21/1 -> Mux2/2
  Reshape 9x1->3x3/1 -> DCMbe/1
  23/1 -> Mux2/8
  33/1 -> Mux2/9
  22/1 -> Mux2/5
  32/1 -> Mux2/6
  phi theta psi/1 -> 23/1, 33/1, 13/1, 32/1, 22/1, 12/1, 31/1, 21/1, 11/1

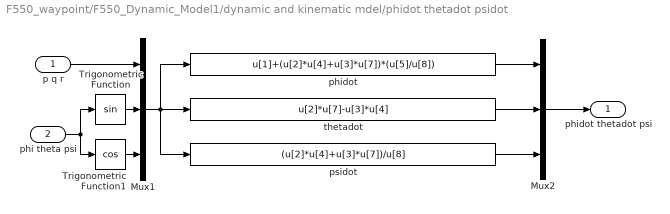
== system F550_waypoint/F550_Dynamic_Model1/dynamic and kinematic mdel/phidot thetadot psidot ==
  p q r : Inport
  phi theta psi : Inport  Port=2
  Mux1 : Mux  Inputs=[3 3 3]
  Mux2 : Mux  Inputs=3
  Trigonometric Function : Trigonometry
  Trigonometric Function1 : Trigonometry  Operator=cos
  phidot : Fcn  Expr=u[1]+(u[2]*u[4]+u[3]*u[7])*(u[5]/u[8])
  psidot : Fcn  Expr=(u[2]*u[4]+u[3]*u[7])/u[8]
  thetadot : Fcn  Expr=u[2]*u[7]-u[3]*u[4]
  phidot thetadot psi : Outport  InitialOutput=0  VectorParamsAs1DForOutWhenUnconnected=off
  wires:
  Trigonometric Function1/1 -> Mux1/3
  Trigonometric Function/1 -> Mux1/2
  Mux2/1 -> phidot thetadot psi/1
  phidot/1 -> Mux2/1
  thetadot/1 -> Mux2/2
  psidot/1 -> Mux2/3
  phi theta psi/1 -> Trigonometric Function1/1, Trigonometric Function/1
  p q r/1 -> Mux1/1
  Mux1/1 -> thetadot/1, phidot/1, psidot/1

== system F550_waypoint/F550_Dynamic_Model1/Motor Model/MotorNonlinearDynamic1/Motor_Dynamics (1st order) ==
  note: radps_dot = (radps_cmd-radps)/Tm
      | or
      | radps/radps_cmd = 1/(Tm*s +1)
  motor_radps_cmd : Inport
  motor_radps0 : Inport  Port=2
  Add : Sum  Inputs=|+-
  Gain : Gain  Gain=1/motorTm
  Integrator : Integrator  InitialConditionSource=external
  motor_radps : Outport  VectorParamsAs1DForOutWhenUnconnected=off
  wires:
  Add/1 -> Gain/1
  motor_radps0/1 -> Integrator/2
  motor_radps_cmd/1 -> Add/1
  Gain/1 -> Integrator/1  "rads_dot"
  Integrator/1 -> Add/2, motor_radps/1  "radps"

== system F550_waypoint/F550_Dynamic_Model1/Motor Model/MotorNonlinearDynamic2/Motor_Dynamics (1st order) ==
  note: radps_dot = (radps_cmd-radps)/Tm
      | or
      | radps/radps_cmd = 1/(Tm*s +1)
  motor_radps_cmd : Inport
  motor_radps0 : Inport  Port=2
  Add : Sum  Inputs=|+-
  Gain : Gain  Gain=1/motorTm
  Integrator : Integrator  InitialConditionSource=external
  motor_radps : Outport  VectorParamsAs1DForOutWhenUnconnected=off
  wires:
  Integrator/1 -> motor_radps/1, Add/2  "radps"
  Gain/1 -> Integrator/1  "rads_dot"
  motor_radps_cmd/1 -> Add/1
  motor_radps0/1 -> Integrator/2
  Add/1 -> Gain/1

== system F550_waypoint/F550_Dynamic_Model1/Motor Model/MotorNonlinearDynamic3/Motor_Dynamics (1st order) ==
  note: radps_dot = (radps_cmd-radps)/Tm
      | or
      | radps/radps_cmd = 1/(Tm*s +1)
  motor_radps_cmd : Inport
  motor_radps0 : Inport  Port=2
  Add : Sum  Inputs=|+-
  Gain : Gain  Gain=1/motorTm
  Integrator : Integrator  InitialConditionSource=external
  motor_radps : Outport  VectorParamsAs1DForOutWhenUnconnected=off
  wires:
  Add/1 -> Gain/1
  motor_radps0/1 -> Integrator/2
  motor_radps_cmd/1 -> Add/1
  Gain/1 -> Integrator/1  "rads_dot"
  Integrator/1 -> Add/2, motor_radps/1  "radps"

== system F550_waypoint/F550_Dynamic_Model1/Motor Model/MotorNonlinearDynamic4/Motor_Dynamics (1st order) ==
  note: radps_dot = (radps_cmd-radps)/Tm
      | or
      | radps/radps_cmd = 1/(Tm*s +1)
  motor_radps_cmd : Inport
  motor_radps0 : Inport  Port=2
  Add : Sum  Inputs=|+-
  Gain : Gain  Gain=1/motorTm
  Integrator : Integrator  InitialConditionSource=external
  motor_radps : Outport  VectorParamsAs1DForOutWhenUnconnected=off
  wires:
  Integrator/1 -> motor_radps/1, Add/2  "radps"
  Gain/1 -> Integrator/1  "rads_dot"
  motor_radps_cmd/1 -> Add/1
  motor_radps0/1 -> Integrator/2
  Add/1 -> Gain/1

== system F550_waypoint/F550_Dynamic_Model1/Motor Model/MotorNonlinearDynamic5/Motor_Dynamics (1st order) ==
  note: radps_dot = (radps_cmd-radps)/Tm
      | or
      | radps/radps_cmd = 1/(Tm*s +1)
  motor_radps_cmd : Inport
  motor_radps0 : Inport  Port=2
  Add : Sum  Inputs=|+-
  Gain : Gain  Gain=1/motorTm
  Integrator : Integrator  InitialConditionSource=external
  motor_radps : Outport  VectorParamsAs1DForOutWhenUnconnected=off
  wires:
  Integrator/1 -> motor_radps/1, Add/2  "radps"
  Gain/1 -> Integrator/1  "rads_dot"
  motor_radps_cmd/1 -> Add/1
  motor_radps0/1 -> Integrator/2
  Add/1 -> Gain/1

== system F550_waypoint/F550_Dynamic_Model1/Motor Model/MotorNonlinearDynamic6/Motor_Dynamics (1st order) ==
  note: radps_dot = (radps_cmd-radps)/Tm
      | or
      | radps/radps_cmd = 1/(Tm*s +1)
  motor_radps_cmd : Inport
  motor_radps0 : Inport  Port=2
  Add : Sum  Inputs=|+-
  Gain : Gain  Gain=1/motorTm
  Integrator : Integrator  InitialConditionSource=external
  motor_radps : Outport  VectorParamsAs1DForOutWhenUnconnected=off
  wires:
  Integrator/1 -> motor_radps/1, Add/2  "radps"
  Gain/1 -> Integrator/1  "rads_dot"
  motor_radps_cmd/1 -> Add/1
  motor_radps0/1 -> Integrator/2
  Add/1 -> Gain/1

== matlab function F550_waypoint/waypoint guidance ==
  data: alt_ref output; u_ref output; pn input; psi_ref output; pe input; wp_north input; wp_east input; wp_alt input; wp_u input; prev_wpt_idx input; curr_wpt_idx output
function [alt_ref,u_ref,psi_ref,curr_wpt_idx] = waypoint_cmd(pn,pe,wp_north,wp_east,wp_alt,wp_u,prev_wpt_idx)

% pn       =  Vehicle North position (m)
% pe       =  Vehicle East  position (m)
% wp_north = Waypoint North position (m) 
% wp_east  = Waypoint East  position (m) 
% wp_alt   = Waypoint altitude (m) 
% wp_u     = Waypoint forward speed (m)  
% prev_wpt_idx = Previous waypoint index
% curr_wpt_idx = Current waypoint index
 
dist_to_wpt = sqrt((pn-wp_north(prev_wpt_idx))^2 + (pe-wp_east(prev_wpt_idx))^2);

no_wp=length(wp_north);
if(dist_to_wpt <=5)
    curr_wpt_idx = prev_wpt_idx + 1;
    if (curr_wpt_idx > no_wp)
        curr_wpt_idx = 1;
    end
else
    curr_wpt_idx = prev_wpt_idx;    
end

n_diff = wp_north(curr_wpt_idx) - pn;
e_diff = wp_east(curr_wpt_idx) - pe;

psi_ref = atan2(e_diff, n_diff);

alt_ref = wp_alt(curr_wpt_idx);
u_ref   = wp_u(curr_wpt_idx);

== matlab function F550_waypoint/HeadingController/MATLAB Function2 ==
  data: psi input; psi_mod output
function psi_mod = wrapToPi(psi)

psi_mod = mod(psi + pi, 2*pi) - pi;

== matlab function F550_waypoint/F550_Dynamic_Model1/Aero Force and Moment ==
  data: Fa output; Ma output; wb input; Vb input; Cd input; Cmd input; dz_cg input
function [Fa,Ma] = fcn(wb,Vb,Cd,Cmd,dz_cg)

 Fa = -Cd*Vb.*abs(Vb);         % Careful for the definition of Cd

 Md = -Cmd.*wb.*abs(wb);       % aerodynamic damping moment
  
 Mfd= [Fa(2)*dz_cg
      -Fa(1)*dz_cg
       0];

 Ma = Mfd + Md;
 
end

== matlab function F550_waypoint/F550_Dynamic_Model1/F450 Quadcopter Prop Force and Moment1 ==
  data: w input; R input; Cm input; Ct input; Fprop output; Mprop output; wb input; Jrp input
function [Fprop, Mprop] = fcn(w, R, Cm, Ct, wb, Jrp)

 %  Obtain the force and torque acting on the body. 
 %  The airframe of the quadrotor is as follows:
 %  3↓   1↑
 %    \ /
 %    / \
 %  2↑   4↓
 %  ↑ stands for counterclockwise and ↓stands for clockwise.
 
 % Input：
 %  w: motor speed，unit：rad/s
 %  R: body radius(m)
 %  Cm: torque coefficient
 %  Ct: thrust coefficient
 %  wb: angular velocity in the body coordinate system
 %  Jrp:  moment of inertia of motor rotor + propeller

 % Output:
 %  Fprop: force vector from prop
 %  Mprop: aerodynamic damping moment + gyro moment

 
 F_prop = Ct*(w.^2);      % Force from each prop
 M_prop = Cm*(w.^2);      % Torque magnitude from each prop

 Fprop = [0; 0; -sum(F_prop)];

 d=sin(pi/4)*R;
 Mp= [ d*F_prop'*[-1;  1;  1; -1]
       d*F_prop'*[ 1; -1;  1; -1]
         M_prop'*[ 1;  1; -1; -1] ];

% gyro moment
 M_gyro   = [Jrp*wb(2)*( w(1) + w(2) - w(3) - w(4));  
             Jrp*wb(1)*(-w(1) - w(2) + w(3) + w(4));
             0];

 Mprop = Mp + M_gyro;

end

== matlab function F550_waypoint/F550_Dynamic_Model1/F550 Hexacopter Prop Force and Moment ==
  data: w input; L input; Cm input; Ct input; Fprop output; Mprop output; wb input; Jrp input
function [Fprop, Mprop] = fcn(w, L, Cm, Ct, wb, Jrp)

 % Body Frame : NED Coordinate
 % X-axis : Heading, Y-axis : Right wing, Z-axis : Down

 %  Obtain the force and torque acting on the body. 
 %  The airframe of the hexarotor is as follows: PX4 Hexacopter Configuration
 %     3↓   5↑
 %      \  /
 %   2↑--  -- 1↓
 %      /  \
 %     6↓   4↑
 %  ↑ stands for counterclockwise and ↓stands for clockwise.


 % Input：
 %  w: motor speed，unit：rad/s
 %  L: Arm Length (m) - In case of F550 R = 0.275 m
 %  Cm: torque coefficient
 %  Ct: thrust coefficient
 %  wb: angular velocity in the body coordinate system
 %  Jrp:  moment of inertia of motor rotor + propeller

 % Output:
 %  Fprop: force vector from prop
 %  Mprop: aerodynamic damping moment + gyro moment
        
        % Legacy Code - From F450 Quadcopter 
        %  F_prop = Ct*(w.^2);      % Force from each prop
        %  M_prop = Cm*(w.^2);      % Torque magnitude from each prop
        % 
        %  Fprop = [0; 0; -sum(F_prop)];
        % 
        %  d=sin(pi/4)*R;
        %  Mp= [ d*F_prop'*[-1;  1;  1; -1]
        %        d*F_prop'*[ 1; -1;  1; -1]
        %          M_prop'*[ 1;  1; -1; -1] ];
        % 
        % % gyro moment
        %  M_gyro   = [Jrp*wb(2)*( w(1) + w(2) - w(3) - w(4));  
        %              Jrp*wb(1)*(-w(1) - w(2) + w(3) + w(4));
        %              0];
        % 
        %  Mprop = Mp + M_gyro;
    
    % 로터 회전수에 따른 추력 및 모멘트
    F_prop = Ct * (w.^2);
    M_prop = Cm * (w.^2);
    
    % 프로펠러에 의한 힘 
    Fprop = [0; 0; -sum(F_prop)];
    
    % 로터에 추력/회전에 의해 기체에 작용하는 모멘트
    Mp = [ F_prop'*[-L; L; 0.5*L; -0.5*L; -0.5*L; 0.5*L]
           F_prop'*[0; 0; sqrt(3)/2*L; -sqrt(3)/2*L; sqrt(3)/2*L; -sqrt(3)/2*L]
           M_prop'*[-1; 1; -1; 1; -1; 1;]
         ];
    
    % 동체 회전에 의해 회전하는 프롭에 작용하는 모멘트
    M_gyro = [Jrp*wb(2)*( -w(1)+w(2)-w(3)+w(4)-w(5)+w(6) );
              -Jrp*wb(1)*( -w(1)+w(2)-w(3)+w(4)-w(5)+w(6));
              0;
        ];
    
    Mprop = Mp + M_gyro;
end
